simulink model "W2Q4"  (R2020b)
settings: Solver=VariableStepAuto  StartTime=0.0  StopTime=100  RelTol=1e-3
values from neighbouring files (symbols this model uses):
  b = 3.5077E-6    (= 3.5077e-06)    [variables.m]
  J = 3.2284E-6    (= 3.2284e-06)    [variables.m]
  K = 0.0274    [variables.m]
  kd = 0.5    [variables.m]
  ki = 5000    [variables.m]
  kp = 100    [variables.m]
  L = 2.75E-6    (= 2.75e-06)    [variables.m]
  n = 120000    [variables.m]
  R = 4    [variables.m]
settings Model: Creator=VIVEK  LastModifiedBy=VIVEK

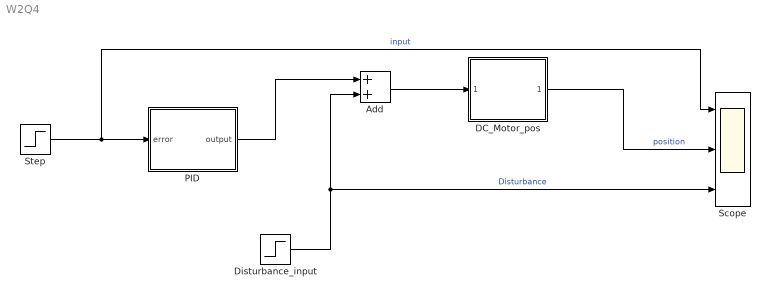
== system W2Q4 ==
  Add : Sum
  DC_Motor_pos : Subsystem
  Disturbance_input : Step  Time=0.06  SampleTime=0
  PID : Subsystem
  Scope : Scope  NumInputPorts=3
  Step : Step  SampleTime=0
  wires:
  Add/1 -> DC_Motor_pos/1(Voltage)
  Step/1 -> Scope/1, PID/1(error)  "input"
  PID/1(output) -> Add/1
  Disturbance_input/1 -> Scope/3, Add/2  "Disturbance"
  DC_Motor_pos/1(Position) -> Scope/2  "position"

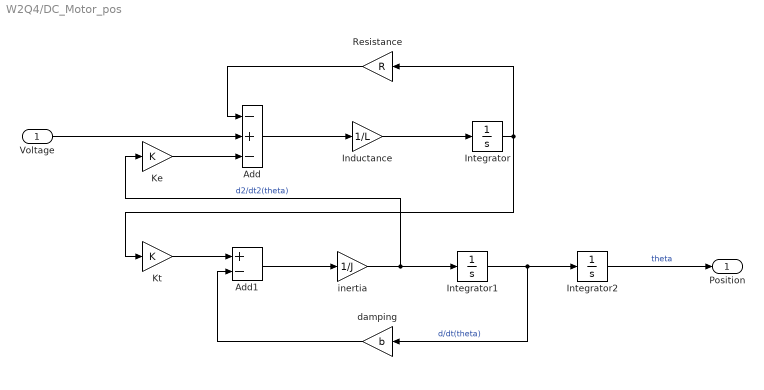
== system W2Q4/DC_Motor_pos ==
  Voltage : Inport
  Add : Sum  Inputs=-+-
  Add1 : Sum  Inputs=+-
  Inductance : Gain  Gain=1/L
  Integrator : Integrator
  Integrator1 : Integrator
  Integrator2 : Integrator
  Ke : Gain  Gain=K
  Kt : Gain  Gain=K
  Resistance : Gain  Gain=R
  damping : Gain  Gain=b
  inertia : Gain  Gain=1/J
  Position : Outport
  wires:
  Kt/1 -> Add1/1
  Inductance/1 -> Integrator/1
  Resistance/1 -> Add/1
  damping/1 -> Add1/2
  inertia/1 -> Ke/1, Integrator1/1  "d2/dt2(theta)"
  Integrator/1 -> Resistance/1, Kt/1
  Integrator1/1 -> damping/1, Integrator2/1  "d/dt(theta)"
  Ke/1 -> Add/3
  Add1/1 -> inertia/1
  Add/1 -> Inductance/1
  Voltage/1 -> Add/2
  Integrator2/1 -> Position/1  "theta"

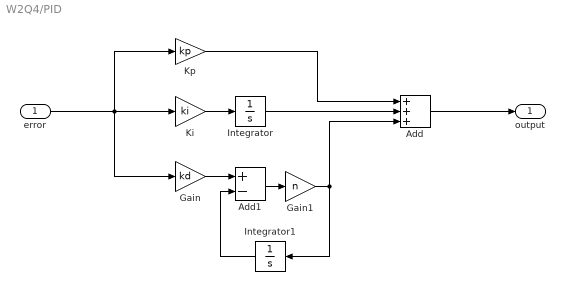
== system W2Q4/PID ==
  error : Inport
  Add : Sum  Inputs=+++
  Add1 : Sum  Inputs=+-
  Gain : Gain  Gain=kd
  Gain1 : Gain  Gain=n
  Integrator : Integrator
  Integrator1 : Integrator
  Ki : Gain  Gain=ki
  Kp : Gain  Gain=kp
  output : Outport
  wires:
  Integrator/1 -> Add/2
  Gain1/1 -> Add/3, Integrator1/1
  Kp/1 -> Add/1
  Add/1 -> output/1
  Add1/1 -> Gain1/1
  error/1 -> Gain/1, Ki/1, Kp/1
  Integrator1/1 -> Add1/2
  Ki/1 -> Integrator/1
  Gain/1 -> Add1/1
